simulink model "DQsymRLC"  (R2024a)
settings: Solver=FixedStepDiscrete  StartTime=0.0  StopTime=1  FixedStep=Ts  RelTol=1e-3
StartFcn:
  | tic
StopFcn:
  | toc
values from neighbouring files (symbols this model uses):
  f = 50    [RLC.m]
  L_lo = 0.002    [RLC.m]
  L_src = 0.00222    [RLC.m]
  N = 5    [RLC.m]
  R_lo = 50    [RLC.m]
  R_src = 0.1    [RLC.m]
  Srlc =     [Srlc.mat]
  Ts = 20e-6    (= 2e-05)    [RLC.m]
  Vnom_prim = 240e3    (= 240000)    [RLC.m]
undefined symbols (not defined in the file or in its folder): S
libraries: DQsym_Lib x4, spsControlledVoltageSourceLib x3, spsGroundLib x2, spsThreePhaseVIMeasurementLib x1, spsThreePhaseParallelRLCBranchLib x1, spsThreePhaseSeriesRLCBranchLib x1, spspowerguiLib x1
settings Model: SimulationMode=accelerator  Creator=The MathWorks, Inc.  LastModifiedBy=salsarayreh
settings SolverCC: AlgebraicLoopSolver=TrustRegion
settings DataIOCC: SaveFormat=StructureWithTime  SaveOutput=off  DSMLogging=off  SaveTime=off  ReturnWorkspaceOutputs=off
settings OptimizationCC: ReuseModelBlockBuffer=off  ExpressionDepthLimit=2147483647  LifeSpan=inf
settings DebuggingCC: UnderspecifiedInitializationDetection=Classic  MergeDetectMultiDrivingBlocksExec=none  SolverPrmCheckMsg=warning  FcnCallInpInsideContextMsg=warning  UnconnectedInputMsg=warning  UnconnectedOutputMsg=warning  UnconnectedLineMsg=warning  AllowSymbolicDim=off  StateNameClashWarn=warning  SFUnexpectedBacktrackingDiag=warning  SFNoUnconditionalDefaultTransitionDiag=warning  SFExecutionAtInitializationDiag=none  ArithmeticOperatorsInVariantConditions=warning
settings HardwareCC: ProdBitPerPointer=32  ProdBitPerSizeT=32  ProdBitPerPtrDiffT=32  ProdLargestAtomicFloat=None  ProdIntDivRoundTo=Undefined  ProdEndianess=Unspecified  ProdWordSize=32  ProdHWDeviceType=32-bit Generic
settings ModelReferenceCC: EnableRefExpFcnMdlSchedulingChecks=on  PropagateSignalLabelsOutOfModel=off
settings SFSimCC: SimUseLocalCustomCode=off  CustomCodeUndefinedFunction=UseInterfaceOnly
settings RTWCC: RTWUseLocalCustomCode=off  GPUComputeCapability=3.5
settings CodeAppCC: StateflowObjectComments=on
settings GRTTargetCC: TargetLangStandard=C89/C90 (ANSI)  CombineOutputUpdateFcns=off  GRTInterface=on
settings ConfigComp: CovMetricSettings=dw  CovSaveCumulativeToWorkspaceVar=on  CovSaveSingleToWorkspaceVar=on  CovExternalEMLEnable=off
settings SimscapeCC: SimscapeNormalizeSystem=off

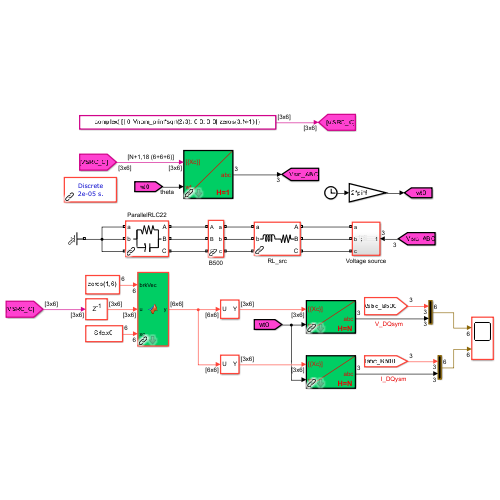
[thumbnail: Simulink's stored preview of the top-level diagram]
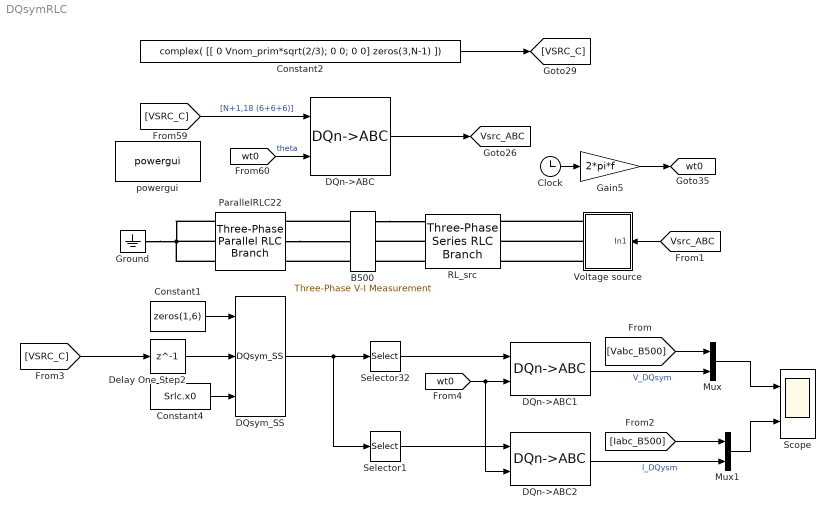
== system DQsymRLC ==
  B500 : spsThreePhaseVIMeasurementLib/Three-Phase V-I Measurement  VoltageMeasurement=phase-to-ground  SetLabelV=on  LabelV=Vabc_B500  Vpu=off  VpuLL=off  CurrentMeasurement=yes  SetLabelI=on  LabelI=Iabc_B500  Ipu=off  Pbase=100e6  Vbase=500e3  OutputType=Complex  PhasorSimulation=off  PSBequivalent=0
  Clock : Clock
  Constant1 : Constant  Value=zeros(1,6)  SampleTime=-1
  Constant2 : Constant  Value=complex( [[ 0 Vnom_prim*sqrt(2/3); 0 0; 0 0] zeros(3,N-1) ])
  Constant4 : Constant  Value=Srlc.x0  SampleTime=-1
  DQn->ABC : DQsym_Lib/DQn->ABC  N=1
      settings: SourceProductName=DQsym Library
  DQn->ABC1 : DQsym_Lib/DQn->ABC  N=N
      settings: SourceProductName=DQsym Library
  DQn->ABC2 : DQsym_Lib/DQn->ABC  N=N
      settings: SourceProductName=DQsym Library
  DQsym_SS : DQsym_Lib/DQsym_SS  Ad=Srlc.A  Bd=Srlc.B  Cd=Srlc.C  Dd=Srlc.D  swOnRes=1e-3*ones(1,6)  swOffRes=1e6*ones(1,6)  swType=ones(1,6)  dt=2e-5  nrSWvec=6
      settings: SourceProductName=DQsym Library
  Delay One Step2 : Delay  DelayLength=1  SampleTime=Ts
  Gain5 : Gain  Gain=2*pi*f
  Ground : spsGroundLib/Ground  LConnTagsString=a
  Mux : Mux  Inputs=2
  Mux1 : Mux  Inputs=2
  ParallelRLC22 : spsThreePhaseParallelRLCBranchLib/Three-Phase Parallel RLC Branch  LConnTagsString=A|B|C  RConnTagsString=A|B|C  BranchType=RC  Resistance=R_lo  Inductance=1e-3  Capacitance=L_lo  Measurements=Branch voltages
  RL_src : spsThreePhaseSeriesRLCBranchLib/Three-Phase Series RLC Branch  LConnTagsString=A|B|C  RConnTagsString=A|B|C  BranchType=RL  Resistance=R_src  Inductance=L_src  Capacitance=1/(0.55*0.080*(500e3^2/100e6))/(2*pi*60)  Measurements=Branch voltages
  Scope : Scope  NumInputPorts=2
  Selector1 : Selector  NumberOfDimensions=2  InputPortWidth=size(S.C,1)  IndexOptions=Index vector (dialog),Select all  Indices=4:6,1  OutputSizes=1,1
  Selector32 : Selector  NumberOfDimensions=2  InputPortWidth=size(S.C,1)  IndexOptions=Index vector (dialog),Select all  Indices=1:3,1  OutputSizes=1,1
  Voltage source : Subsystem
  powergui : spspowerguiLib/powergui  Priority=1  SimulationMode=Discrete  SampleTime=Ts  frequency=60  Iterations=50  frequencyindice=0  Pbase=100e6  ErrMax=1e-4  UnitsV=kV  UnitsW=MW  buscounter=0  FunctionMessages=off  echomessages=off  EnableUseOfTLC=off  CurrentSourceSwitches=off  DisableSnubberDevices=off  DisableRonSwitches=off  DisableVfSwitches=off  DisplayEquations=off  AutomaticDiscreteSolvers=off  SolverType=Tustin/Backward Euler (TBE)  Interpol=off  ExternalGateDelay=off  methode=off  Ts=10  x0status=blocks  SPID=off  SwTol=0  HookPort=off  NonlinearTolerance=1e-4  nMaxIteration=100  ContinueOnMaxIteration=off  RestoreLinks=warning  ResistiveCurrentMeasurement=off  Frange=[0:2:500]  Ylog=off  Xlog=on  ShowGrid=off  save=off  variable=ZData  structure=VIprim  ZoomFFT=on  StartTime=0.15  cycles=2  DisplayStyle=1  fundamental=50  FreqAxis=on  MaxFrequency=1000  frequencyindicesteady=1  RmsSteady=1  display=off
  tag scope: Vsrc_ABC=global, wt0=global
  wires:
  Clock/1 -> Gain5/1
  Gain5/1 -> [wt0]
  DQn->ABC/1 -> [Vsrc_ABC]
  [wt0] -> DQn->ABC/2  "theta"
  Constant2/1 -> [VSRC_C]
  [VSRC_C] -> DQn->ABC/1  "[N+1,18 (6+6+6)]"
  [Vsrc_ABC] -> Voltage source/1(In1)
  [Iabc_B500] -> Mux1/1
  Selector32/1 -> DQn->ABC1/1
  Selector1/1 -> DQn->ABC2/1
  [wt0] -> DQn->ABC2/2, DQn->ABC1/2
  Mux/1 -> Scope/1
  DQn->ABC2/1 -> Mux1/2  "I_DQysm"
  Mux1/1 -> Scope/2
  [Vabc_B500] -> Mux/1
  DQn->ABC1/1 -> Mux/2  "V_DQsym"
  DQsym_SS/1 -> Selector1/1, Selector32/1
  [VSRC_C] -> Delay One Step2/1
  Constant4/1 -> DQsym_SS/3
  Delay One Step2/1 -> DQsym_SS/2
  Constant1/1 -> DQsym_SS/1
  connections:
  B500/LConn3 -- ParallelRLC22/LConn3
  ParallelRLC22/LConn2 -- B500/LConn2
  ParallelRLC22/RConn1 -- ParallelRLC22/RConn2 -- Ground/LConn1 -- ParallelRLC22/RConn3
  B500/LConn1 -- ParallelRLC22/LConn1
  Voltage source/RConn3 -- RL_src/LConn3
  B500/RConn1 -- RL_src/RConn1
  Voltage source/RConn2 -- RL_src/LConn2
  Voltage source/RConn1 -- RL_src/LConn1
  RL_src/RConn2 -- B500/RConn2
  RL_src/RConn3 -- B500/RConn3

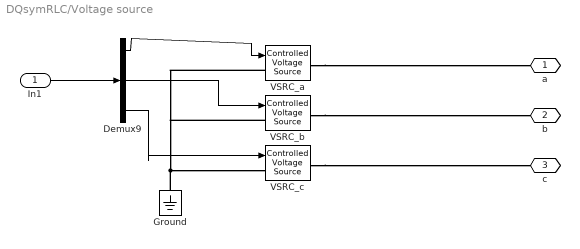
== system DQsymRLC/Voltage source ==
  In1 : Inport
  Demux9 : Demux  Outputs=3
  Ground : spsGroundLib/Ground  LConnTagsString=a
  VSRC_a : spsControlledVoltageSourceLib/Controlled Voltage Source  Initialize=on  Source_Type=AC  Amplitude=0  Phase=0  Frequency=0  Measurements=None
  VSRC_b : spsControlledVoltageSourceLib/Controlled Voltage Source  Initialize=on  Source_Type=AC  Amplitude=0  Phase=0  Frequency=0  Measurements=None
  VSRC_c : spsControlledVoltageSourceLib/Controlled Voltage Source  Initialize=on  Source_Type=AC  Amplitude=0  Phase=0  Frequency=0  Measurements=None
  a : PMIOPort  Side=Right
  b : PMIOPort  Port=2  Side=Right
  c : PMIOPort  Port=3  Side=Right
  wires:
  In1/1 -> Demux9/1
  Demux9/1 -> VSRC_a/1
  Demux9/2 -> VSRC_b/1
  Demux9/3 -> VSRC_c/1
  connections:
  Ground/LConn1 -- VSRC_b/LConn1 -- VSRC_a/LConn1 -- VSRC_c/LConn1
  VSRC_c/RConn1 -- c/RConn1
  VSRC_b/RConn1 -- b/RConn1
  VSRC_a/RConn1 -- a/RConn1
